simulink model "PMSM_realmodel"  (R2022b)
settings: Solver=FixedStepAuto  StartTime=0.0  StopTime=1  FixedStep=1e-6  MaxStep=1e-3  RelTol=1e-3
values from neighbouring files (symbols this model uses):
  a_fw = log(9)/trfw    [emrax_sim.m]
  ba = 2*k^2*(as*J - bm)/(np^2*psi)    [emrax_sim.m]
  bm = 0.008    [emrax_sim.m]
  fsw = 8e3    (= 8000)    [emrax_sim.m]
  I_max = I_base    [emrax_sim.m]
  J = 421e-4    (= 0.0421)    [emrax_sim.m]
  k = 1    [emrax_sim.m]
  ki_d = (ac^2)*Ld    [emrax_sim.m]
  ki_q = (ac^2)*Lq    [emrax_sim.m]
  ki_s = 2*k^2*as^2*J/(np^2*psi)    [emrax_sim.m]
  kp_d = ac*Ld    [emrax_sim.m]
  kp_q = ac*Lq    [emrax_sim.m]
  kp_s = 2*k^2*as*J/(np^2*psi)    [emrax_sim.m]
  Ld = 177*10^(-6)    (= 0.000177)    [emrax_sim.m]
  Lq = 183*10^(-6)    (= 0.000183)    [emrax_sim.m]
  np = 10    [emrax_sim.m]
  Peak_power = 50000    [emrax_sim.m]
  Peak_regen = -1500000    [emrax_sim.m]
  psi = 0.0542*k    (= 0.0542)    [emrax_sim.m]
  Ra_d = ac*Ld-Rs    [emrax_sim.m]
  Ra_q = ac*Lq-Rs    [emrax_sim.m]
  rpm_nom = 5100    [emrax_sim.m]
  Rs = 18e-3    (= 0.018)    [emrax_sim.m]
  u_dc = 550    [emrax_sim.m]
  u_nom = u_dc*k    (= 550)    [emrax_sim.m]
undefined symbols (not defined in the file or in its folder): Icutoff, rc1, rc2, rc3, rc4, rc5
libraries: simulink x9, spsIGBTDiodeLib x6, dspstat3 x3, spsCurrentMeasurementLib x3, spsSeriesRLCBranchLib x3, spsDCVoltageSourceLib x1, spsPermanentMagnetSynchronousMachineLib x1, spsThreePhaseVIMeasurementLib x1, spsMultimeterLib x1, spsTriangleGeneratorLib x1, sps_lib x1
settings Model: Creator=Vaggelis  LastModifiedBy=alexa
settings SolverCC: AlgebraicLoopSolver=TrustRegion
settings DebuggingCC: UnconnectedInputMsg=warning  UnconnectedOutputMsg=warning  UnconnectedLineMsg=warning  ArithmeticOperatorsInVariantConditions=warning
settings ModelReferenceCC: EnableRefExpFcnMdlSchedulingChecks=on
settings SFSimCC: CustomCodeUndefinedFunction=UseInterfaceOnly
settings RTWCC: DLArmComputeVersion=19.05

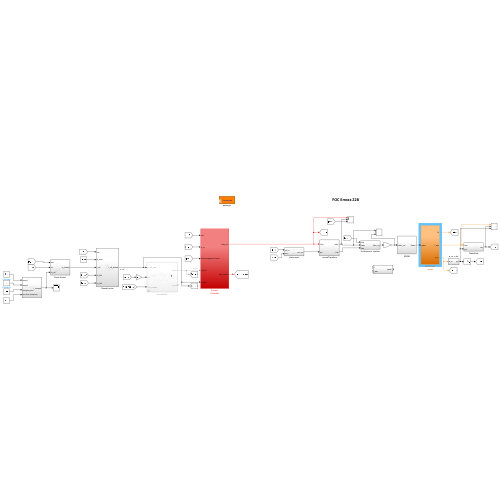
[thumbnail: Simulink's stored preview of the top-level diagram]
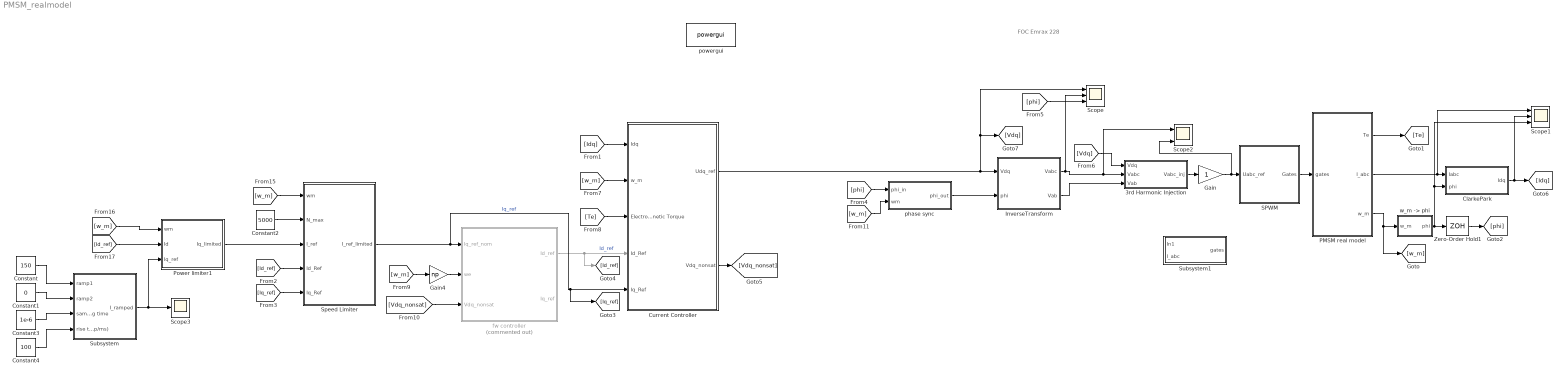
== system PMSM_realmodel ==
  note: FOC Emrax 228
  3rd Harmonic Injection : Subsystem
  ClarkePark : Subsystem
  Constant : Constant  Value=150
  Constant1 : Constant  Value=0
  Constant2 : Constant  Value=5000
  Constant3 : Constant  Value=1e-6
  Constant4 : Constant  Value=100
  Current Controller : Subsystem
  Gain : Gain
  Gain4 : Gain  Gain=np
  InverseTransform : Subsystem
  PMSM real model : Subsystem
  Power limiter1 : Subsystem
  SPWM : Subsystem
  Scope : Scope  NumInputPorts=3
  Scope1 : Scope  NumInputPorts=3
  Scope2 : Scope  NumInputPorts=3
  Scope3 : Scope
  Speed Limiter : Subsystem
  Subsystem : Subsystem
  Subsystem1 : Subsystem
  Zero-Order Hold1 : ZeroOrderHold  SampleTime=62e-6
  fw controller : Subsystem  Commented=on
  phase sync : Subsystem
  powergui : sps_lib/powergui  Priority=1  SimulationMode=Continuous  SampleTime=50e-6  frequency=60  Iterations=50  frequencyindice=0  Pbase=100e6  ErrMax=1e-4  UnitsV=kV  UnitsW=MW  buscounter=0  FunctionMessages=off  echomessages=off  EnableUseOfTLC=off  CurrentSourceSwitches=off  DisableSnubberDevices=off  DisableRonSwitches=off  DisableVfSwitches=off  DisplayEquations=off  AutomaticDiscreteSolvers=off  SolverType=Tustin/Backward Euler (TBE)  Interpol=off  ExternalGateDelay=off  methode=off  Ts=100  x0status=blocks  SPID=on  SwTol=0  HookPort=off  NonlinearTolerance=0  nMaxIteration=15  ContinueOnMaxIteration=off  RestoreLinks=warning  ResistiveCurrentMeasurement=off  Frange=[0:2:500]  Ylog=off  Xlog=on  ShowGrid=off  save=off  variable=ZData  structure=0  ZoomFFT=off  StartTime=0.0  cycles=1  DisplayStyle=1  fundamental=60  FreqAxis=off  MaxFrequency=1000  frequencyindicesteady=1  RmsSteady=1  display=off
  "w_m -> phi" : Subsystem
  wires:
  PMSM real model/3(w_m) -> [w_m], "w_m -> phi"/1(w_m)
  PMSM real model/1(Te) -> [Te]
  SPWM/1(Gates) -> PMSM real model/1("gates ")
  [Te] -> Current Controller/3(Electromagnetic Torque)
  Power limiter1/1(Iq_limited) -> Speed Limiter/3(I_ref)
  [w_m] -> Current Controller/2(w_m)
  [Iq_ref] -> Speed Limiter/5(Iq_Ref)
  [w_m] -> Gain4/1
  Constant2/1 -> Speed Limiter/2(N_max)
  [Id_ref] -> Power limiter1/2(Id)
  [Idq] -> Current Controller/1(Idq)
  [w_m] -> Power limiter1/1(wm)
  fw controller/1(Id_ref) -> [Id_ref], Current Controller/4(Id_Ref)  "Id_ref"
  Gain4/1 -> fw controller/2(we)
  [w_m] -> Speed Limiter/1(wm)
  Current Controller/2(Vdq_nonsat) -> [Vdq_nonsat]
  [Vdq_nonsat] -> fw controller/3(Vdq_nonsat)
  [Id_ref] -> Speed Limiter/4(Id_Ref)
  "w_m -> phi"/1(phi) -> ClarkePark/2(phi), Scope1/3, Zero-Order Hold1/1
  PMSM real model/2(I_abc) -> Scope1/1, ClarkePark/1(Iabc)
  ClarkePark/1(Idq) -> Scope1/2, [Idq]
  [phi] -> Scope/3
  Current Controller/1("Udq_ref ") -> Scope/1, [Vdq], InverseTransform/1(Vdq)
  3rd Harmonic Injection/1(Vabc_inj) -> Gain/1
  InverseTransform/1(Vabc) -> Scope/2, Scope2/1, 3rd Harmonic Injection/2(Vabc)
  [Vdq] -> 3rd Harmonic Injection/1(Vdq)
  InverseTransform/2(Vab) -> 3rd Harmonic Injection/3(Vab)
  Gain/1 -> SPWM/1(Uabc_ref), Scope2/3
  [phi] -> phase sync/1(phi_in)
  [w_m] -> phase sync/2(wm)
  phase sync/1(phi_out) -> InverseTransform/2(phi)
  Subsystem/1(I_ramped) -> Power limiter1/3(Iq_ref), Scope3/1
  Constant/1 -> Subsystem/1(ramp1)
  Constant1/1 -> Subsystem/2(ramp2)
  Constant3/1 -> Subsystem/3(sampling time)
  Constant4/1 -> Subsystem/4(rise time (Amp/ms))
  Zero-Order Hold1/1 -> [phi]
  Speed Limiter/1(I_ref_limited) -> [Iq_ref], Current Controller/5(Iq_Ref), fw controller/1(Iq_ref_nom)  "Iq_ref"

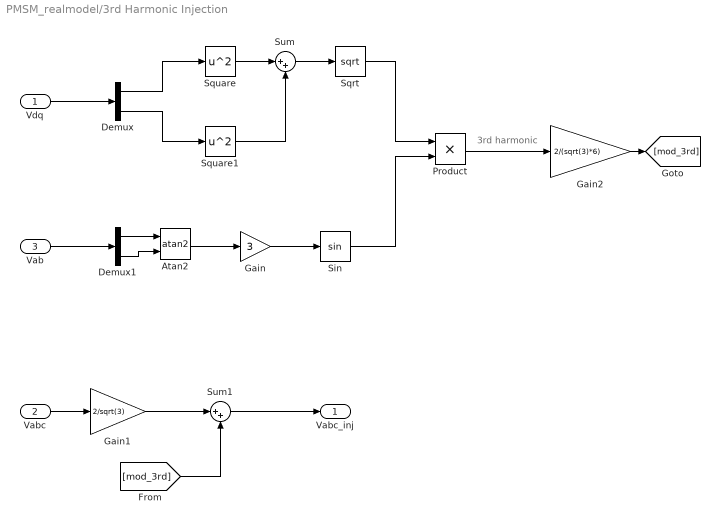
== system PMSM_realmodel/3rd Harmonic Injection ==
  note: 3rd harmonic
  Vdq : Inport
  Vabc : Inport  Port=2
  Vab : Inport  Port=3
  Atan2 : Trigonometry  Operator=atan2
  Demux : Demux  Outputs=2
  Demux1 : Demux  Outputs=2
  Gain : Gain  Gain=3
  Gain1 : Gain  Gain=2/sqrt(3)
  Gain2 : Gain  Gain=2/(sqrt(3)*6)
  Product : Product
  Sin : Trigonometry
  Sqrt : Sqrt
  Square : Math  Operator=square
  Square1 : Math  Operator=square
  Sum : Sum  Inputs=|++
  Sum1 : Sum  Inputs=|++
  Vabc_inj : Outport
  wires:
  Vdq/1 -> Demux/1
  Demux/1 -> Square/1
  Demux/2 -> Square1/1
  Square/1 -> Sum/1
  Square1/1 -> Sum/2
  Sum/1 -> Sqrt/1
  Vab/1 -> Demux1/1
  Demux1/1 -> Atan2/1
  Demux1/2 -> Atan2/2
  Atan2/1 -> Gain/1
  Gain/1 -> Sin/1
  Sqrt/1 -> Product/1
  Sin/1 -> Product/2
  Vabc/1 -> Gain1/1
  Product/1 -> Gain2/1
  Gain2/1 -> [mod_3rd]
  Gain1/1 -> Sum1/1
  [mod_3rd] -> Sum1/2
  Sum1/1 -> Vabc_inj/1

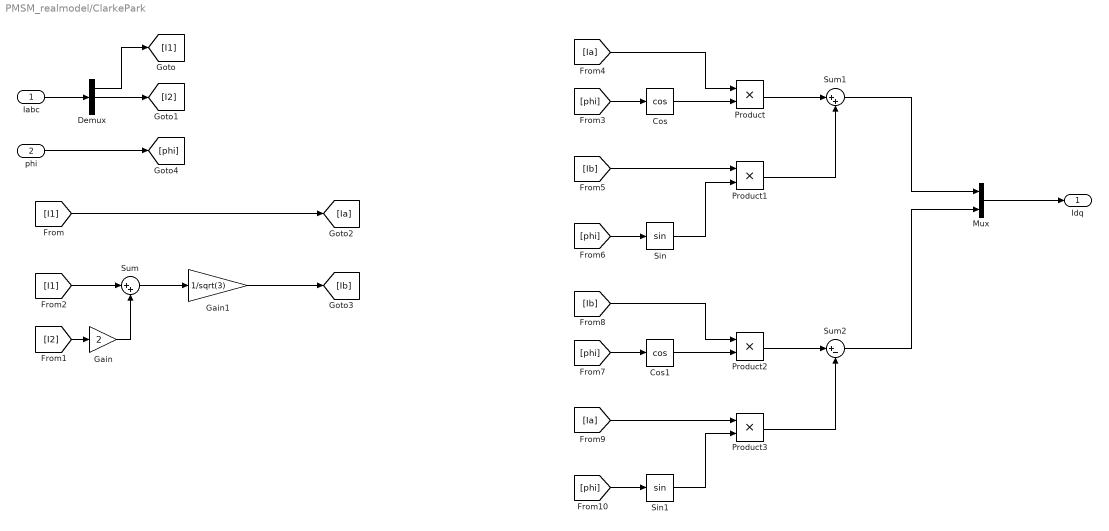
== system PMSM_realmodel/ClarkePark ==
  Iabc : Inport
  phi : Inport  Port=2
  Cos : Trigonometry  Operator=cos
  Cos1 : Trigonometry  Operator=cos
  Demux : Demux  Outputs=3
  Gain : Gain  Gain=2
  Gain1 : Gain  Gain=1/sqrt(3)
  Mux : Mux  Inputs=2
  Product{,1..3} (4 alike) : Product
  Sin : Trigonometry
  Sin1 : Trigonometry
  Sum : Sum  Inputs=|++
  Sum1 : Sum  Inputs=|++
  Sum2 : Sum  Inputs=|+-
  Idq : Outport
  wires:
  Iabc/1 -> Demux/1
  Demux/1 -> [I1]
  Demux/2 -> [I2]
  [I1] -> [Ia]
  [I1] -> Sum/1
  [I2] -> Gain/1
  Gain/1 -> Sum/2
  Sum/1 -> Gain1/1
  Gain1/1 -> [Ib]
  phi/1 -> [phi]
  [phi] -> Cos/1
  Cos/1 -> Product/2
  [Ia] -> Product/1
  Product/1 -> Sum1/1
  [phi] -> Sin/1
  [Ib] -> Product1/1
  Sin/1 -> Product1/2
  Product1/1 -> Sum1/2
  Sum1/1 -> Mux/1
  Mux/1 -> Idq/1
  Product3/1 -> Sum2/2
  Sin1/1 -> Product3/2
  [Ia] -> Product3/1
  [phi] -> Sin1/1
  Product2/1 -> Sum2/1
  [Ib] -> Product2/1
  Cos1/1 -> Product2/2
  [phi] -> Cos1/1
  Sum2/1 -> Mux/2

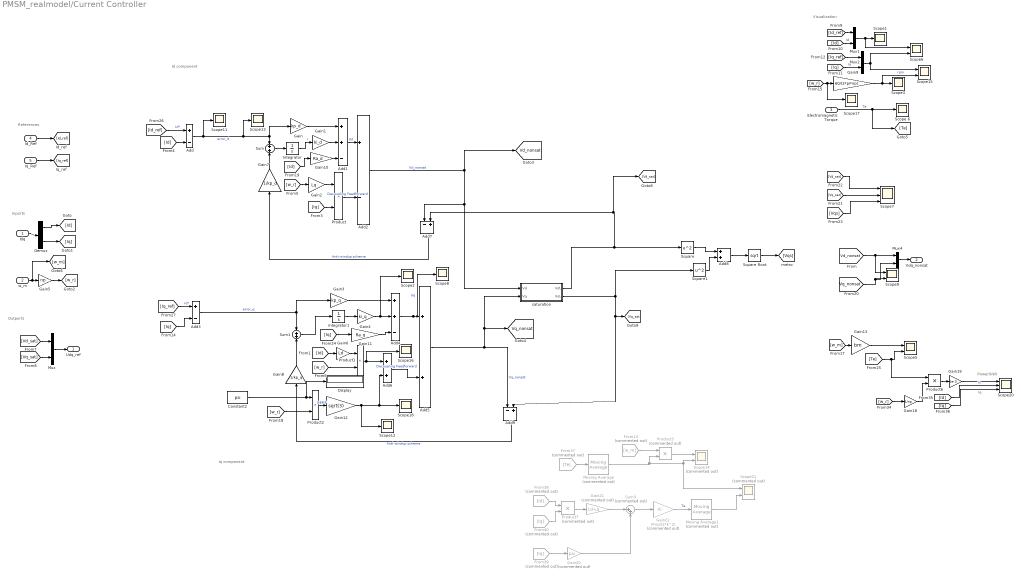
== system PMSM_realmodel/Current Controller ==
  note: References
  note: Id component
  note: Iq component
  note: Inports
  note: Outports
  note: Visualization
  note: Power(kW)
  Idq : Inport
  w_m : Inport  Port=2
  Electromagnetic Torque : Inport  Port=3
  Id_Ref : Inport  Port=4
  Iq_Ref : Inport  Port=5
  Add : Sum  Inputs=+-
  Add1 : Sum  Inputs=++-
  Add2 : Sum  Inputs=+-
  Add3 : Sum  Inputs=+-
  Add4 : Sum  Inputs=++-
  Add5 : Sum
  Add6 : Sum
  Add7 : Sum  Inputs=-+
  Add8 : Sum
  Add9 : Sum  Inputs=-+
  Constant2 : Constant  Value=psi
  Demux : Demux  Outputs=2
  Display : Display
  From13 : From  Commented=on  GotoTag=w_m
  From37 : From  Commented=on  GotoTag=Te
  From38 : From  Commented=on  GotoTag=Id
  From39 : From  Commented=on  GotoTag=Iq
  From40 : From  Commented=on  GotoTag=Iq
  Gain : Gain  Gain=kp_d
  Gain1 : Gain  Gain=ki_d
  Gain10 : Gain  Gain=Ra_d
  Gain11 : Gain  Gain=Ra_q
  Gain12 : Gain  Gain=sqrt(3)
  Gain13 : Gain  Gain=bm
  Gain18 : Gain  Gain=1/np
  Gain19 : Gain  Gain=1e-3
  Gain2 : Gain  Gain=Lq
  Gain20 : Gain  Commented=on  Gain=psi
  Gain21 : Gain  Commented=on  Gain=Ld-Lq
  Gain22 : Gain  Commented=on  Gain=3*np/(2*k^2)
  Gain3 : Gain  Gain=kp_q
  Gain4 : Gain  Gain=ki_q
  Gain5 : Gain  Gain=np
  Gain6 : Gain  Gain=Ld
  Gain7 : Gain  Gain=1/kp_d
  Gain8 : Gain  Gain=1/kp_q
  Gain9 : Gain  Gain=60/(2*pi*np)
  Integrator : Integrator
  Integrator1 : Integrator
  Moving Average : dspstat3/Moving Average  Commented=on  Method=Sliding window  ForgettingFactorPort=off  SpecifyWindowLength=on  WindowLength=40000  OverlapLength=39999  AllowArbitraryInputLength=off  ForgettingFactor=0.9  SimulateUsing=Code generation
  Moving Average1 : dspstat3/Moving Average  Commented=on  Method=Sliding window  ForgettingFactorPort=off  SpecifyWindowLength=on  WindowLength=40000  OverlapLength=39999  AllowArbitraryInputLength=off  ForgettingFactor=0.9  SimulateUsing=Code generation
  Mux{,1..2,4} (4 alike) : Mux  Inputs=2
  Product{,1..2,6} (4 alike) : Product
  Product3 : Product  Commented=on
  Product7 : Product  Commented=on
  Scope 6 : Scope
  Scope{1..3,8,11..13,16..18} (10 alike) : Scope
  Scope14 : Scope  Commented=on  NumInputPorts=2
  Scope{5..6,9,15} (4 alike) : Scope  NumInputPorts=2
  Scope20 : Scope  NumInputPorts=3
  Scope21 : Scope  Commented=on  NumInputPorts=2
  Scope7 : Scope  NumInputPorts=3
  Square : Math  Operator=square
  Square Root : Sqrt
  Square1 : Math  Operator=square
  Sum : Sum
  Sum1 : Sum
  Sum3 : Sum  Commented=on  Inputs=|++
  saturation : Subsystem
  "Udq_ref " : Outport  VectorParamsAs1DForOutWhenUnconnected=off
  Vdq_nonsat : Outport  Port=2
  tag scope: Vd_nonsat=global, Vq_nonsat=global
  wires:
  Gain4/1 -> Scope2/1, Add4/2
  [Id] -> Gain6/1
  Add4/1 -> Scope8/1, Add5/1  "Uq"
  Add1/1 -> Add2/1  "Ud"
  [w_r] -> Gain2/1
  Gain2/1 -> Product/1
  Gain3/1 -> Add4/1
  [Iq] -> Product/2
  Integrator/1 -> Gain1/1  "I"
  Sum/1 -> Integrator/1
  Gain/1 -> Add1/1
  [w_r] -> Product1/2
  Gain6/1 -> Product1/1
  Idq/1 -> Demux/1
  Product/1 -> Add2/2  "Decoupling Feedforward"
  Gain7/1 -> Sum/2
  Add2/1 -> [Vd_nonsat], saturation/1(Vd), Add7/1  "Vd_nonsat"
  Add7/1 -> Gain7/1  "Anti-windup scheme"
  Sum1/1 -> Integrator1/1
  Add5/1 -> Add9/1, saturation/2(Vq), [Vq_nonsat]  "Vq_nonsat"
  Gain8/1 -> Sum1/2
  Add9/1 -> Gain8/1  "Anti-windup scheme"
  Demux/1 -> [Id]
  Demux/2 -> [Iq]
  w_m/1 -> [w_m], Gain5/1
  Gain5/1 -> [w_r]
  [Vd_sat] -> Mux/1
  [Vq_sat] -> Mux/2
  Mux/1 -> "Udq_ref "/1
  [Id] -> Add/2
  Mux1/1 -> Scope6/1, Scope1/1
  [Id_ref] -> Mux1/1
  [Id] -> Mux1/2  "Id"
  [Iq_ref] -> Mux2/1
  [Iq] -> Mux2/2  "Iq"
  [w_r] -> Scope17/1, Gain9/1
  Gain9/1 -> Scope15/2, Scope3/1  "rpm"
  Electromagnetic Torque/1 -> Scope 6/1, [Te]  "Te"
  Product1/1 -> Scope16/1, Add6/1
  Add6/1 -> Add5/2  "Decoupling Feedforward"
  Add/1 -> Scope13/1, Sum/1, Gain/1, Scope11/1  "error_d"
  Add3/1 -> Sum1/1, Gain3/1  "error_q"
  [Iq] -> Add3/2
  Gain1/1 -> Add1/2
  Integrator1/1 -> Gain4/1
  Square1/1 -> Add8/2
  Square/1 -> Add8/1
  Add8/1 -> Square Root/1
  [Vd_nonsat] -> Scope9/1, Mux4/1
  [Vq_nonsat] -> Mux4/2, Scope9/2
  Square Root/1 -> [Vqs]
  [Vd_sat] -> Scope7/1
  [Vq_sat] -> Scope7/2
  [Vqs] -> Scope7/3
  [Id] -> Gain10/1
  [Iq] -> Gain11/1
  Id_Ref/1 -> [Id_ref]
  Iq_Ref/1 -> [Iq_ref]
  Gain13/1 -> Scope5/1
  [Te] -> Product6/1, Scope5/2
  [w_m] -> Gain13/1
  Mux2/1 -> Scope6/2, Scope15/1
  [Id_ref] -> Add/1  "Id*"
  saturation/1(Vd\) -> Square/1, [Vd_sat], Add7/2
  saturation/2(Vq\) -> Square1/1, [Vq_sat], Add9/2
  Gain10/1 -> Add1/3
  Gain11/1 -> Add4/3
  [w_r] -> Product2/2
  Product2/1 -> Gain12/1  "BEMF"
  Mux4/1 -> Vdq_nonsat/1
  [Iq_ref] -> Add3/1  "Id*"
  Gain19/1 -> Scope20/1
  [Iq] -> Scope20/3  "Iq"
  [Id] -> Scope20/2  "Id"
  Gain18/1 -> Product6/2
  Product6/1 -> Gain19/1
  [w_r] -> Gain18/1
  Constant2/1 -> Display/1, Product2/1
  Product3/1 -> Scope14/1
  From13/1 -> Product3/1
  Moving Average/1 -> Scope14/2, Scope21/1, Product3/2
  From37/1 -> Moving Average/1
  From39/1 -> Gain20/1
  Product7/1 -> Gain21/1
  From38/1 -> Product7/1
  From40/1 -> Product7/2
  Gain21/1 -> Sum3/1
  Gain20/1 -> Sum3/2
  Sum3/1 -> Gain22/1
  Gain22/1 -> Moving Average1/1  "Te"
  Moving Average1/1 -> Scope21/2
  Gain12/1 -> Scope12/1, Add6/2, Scope18/1

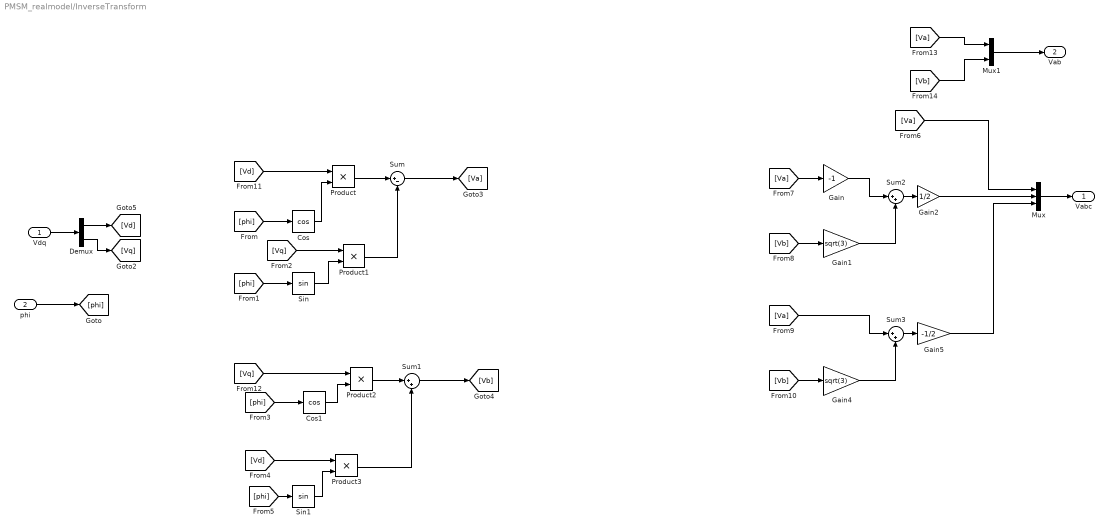
== system PMSM_realmodel/InverseTransform ==
  Vdq : Inport
  phi : Inport  Port=2
  Cos : Trigonometry  Operator=cos
  Cos1 : Trigonometry  Operator=cos
  Demux : Demux  Outputs=2
  Gain : Gain  Gain=-1
  Gain1 : Gain  Gain=sqrt(3)
  Gain2 : Gain  Gain=1/2
  Gain4 : Gain  Gain=sqrt(3)
  Gain5 : Gain  Gain=-1/2
  Mux : Mux  Inputs=3
  Mux1 : Mux  Inputs=2
  Product{,1..3} (4 alike) : Product
  Sin : Trigonometry
  Sin1 : Trigonometry
  Sum : Sum  Inputs=|+-
  Sum1 : Sum  Inputs=|++
  Sum2 : Sum  Inputs=|++
  Sum3 : Sum  Inputs=|++
  Vabc : Outport
  Vab : Outport  Port=2
  wires:
  phi/1 -> [phi]
  [phi] -> Cos/1
  Cos/1 -> Product/2
  Product/1 -> Sum/1
  [phi] -> Sin/1
  [Vq] -> Product1/1
  Sin/1 -> Product1/2
  Product1/1 -> Sum/2
  Cos1/1 -> Product2/2
  [phi] -> Cos1/1
  Product2/1 -> Sum1/1
  Sin1/1 -> Product3/2
  [phi] -> Sin1/1
  [Vd] -> Product3/1
  Product3/1 -> Sum1/2
  Sum/1 -> [Va]
  Sum1/1 -> [Vb]
  [Va] -> Mux/1
  [Va] -> Gain/1
  [Vb] -> Gain1/1
  Gain/1 -> Sum2/1
  Gain1/1 -> Sum2/2
  Sum2/1 -> Gain2/1
  Gain2/1 -> Mux/2
  Sum3/1 -> Gain5/1
  Gain4/1 -> Sum3/2
  [Va] -> Sum3/1
  [Vb] -> Gain4/1
  Vdq/1 -> Demux/1
  Demux/1 -> [Vd]
  Demux/2 -> [Vq]
  [Vd] -> Product/1
  [Vq] -> Product2/1
  Gain5/1 -> Mux/3
  Mux/1 -> Vabc/1
  Mux1/1 -> Vab/1
  [Va] -> Mux1/1
  [Vb] -> Mux1/2

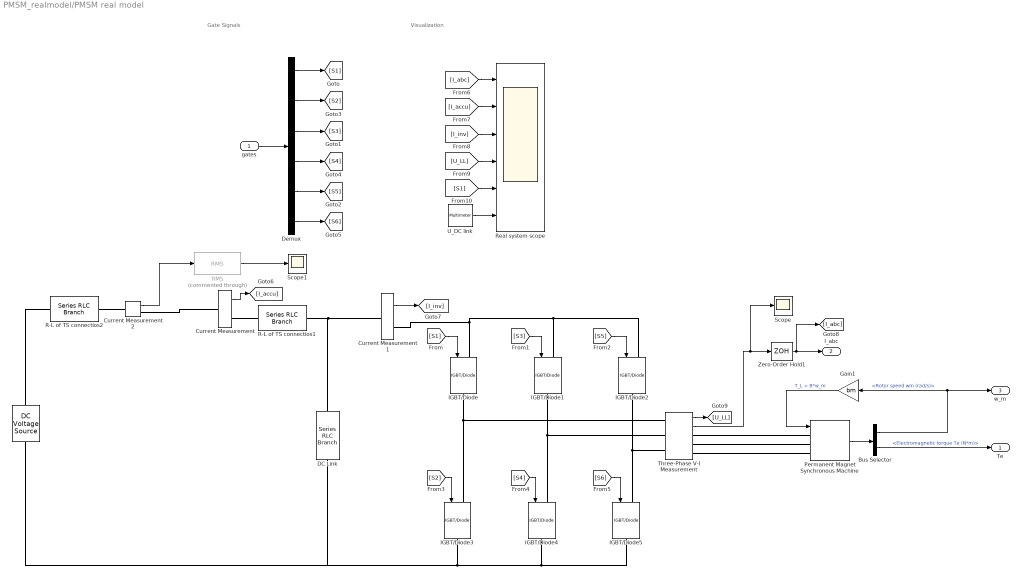
== system PMSM_realmodel/PMSM real model ==
  note: Gate Signals
  note: Visualization
  "gates " : Inport
  " " : spsDCVoltageSourceLib/DC Voltage Source  Description=source block  Amplitude=u_dc  Measurements=None
      settings: AttributesFormatString=\n
  Bus Selector : BusSelector  OutputSignals=Rotor speed wm (rad/s),Electromagnetic torque Te (N*m)
  Current Measurement : spsCurrentMeasurementLib/Current Measurement  PhasorSimulation=off  OutputType=Complex  PSBequivalent=0
  Current Measurement1 : spsCurrentMeasurementLib/Current Measurement  PhasorSimulation=off  OutputType=Complex  PSBequivalent=0
  Current Measurement2 : spsCurrentMeasurementLib/Current Measurement  PhasorSimulation=off  OutputType=Complex  PSBequivalent=0
  DC Link : spsSeriesRLCBranchLib/Series RLC Branch  LConnTagsString=__new0  RConnTagsString=__new0  BranchType=C  Resistance=1  Inductance=1e-3  SetiL0=off  InitialCurrent=0  Capacitance=700e-6  Setx0=off  InitialVoltage=0  Measurements=Branch voltage
  Demux : Demux  Outputs=6
  Gain1 : Gain  Gain=bm
  IGBT/Diode{,1..5} (6 alike) : spsIGBTDiodeLib/IGBT//Diode  Ron=1e-3  Rs=1e5  Cs=inf  Measurements=off
  Permanent Magnet Synchronous Machine : spsPermanentMagnetSynchronousMachineLib/Permanent Magnet Synchronous Machine  NbPhases=3  FluxDistribution=Sinusoidal  RotorType=Salient-pole  MechanicalLoad=Torque Tm  PresetModel=No  ShowDetailedParameters=on  MeasurementBus=off  Resistance=Rs  Inductance=8.5e-3  dqInductances=[Ld Lq]  La=0.00153  MachineConstant=Flux linkage established by magnets (V.s)  Flux=psi  VoltageCst=98.3079  TorqueCst=0.813  Flat=120  Mechanical=[J 0 np 0]  PolePairs=4  InitialConditions=[0,0, 0,0]  InitialConditions5ph=[0 0 0 0 0 0]  RefAngle=Aligned with phase A axis (original Park)  IterativeDiscreteModel=Trapezoidal non iterative  TsBlock=-1  TsPowergui=0
  R-L of TS connectios1 : spsSeriesRLCBranchLib/Series RLC Branch  LConnTagsString=__new0  RConnTagsString=__new0  BranchType=RL  Resistance=20e-4  Inductance=1e-8  SetiL0=off  InitialCurrent=0  Capacitance=300e-6  Setx0=off  InitialVoltage=0  Measurements=None
  R-L of TS connectios2 : spsSeriesRLCBranchLib/Series RLC Branch  LConnTagsString=__new0  RConnTagsString=__new0  BranchType=RL  Resistance=86.4e-3  Inductance=1e-7  SetiL0=off  InitialCurrent=0  Capacitance=300e-6  Setx0=off  InitialVoltage=0  Measurements=None
  RMS : dspstat3/RMS  Commented=through  run=off  directionMode=Each column  dimension=1  InputProcessing=Columns as channels (frame based)  reset_popup=None
  Real system scope : Scope  NumInputPorts=6
  Scope : Scope
  Scope1 : Scope
  Three-Phase V-I Measurement : spsThreePhaseVIMeasurementLib/Three-Phase V-I Measurement  VoltageMeasurement=phase-to-phase  SetLabelV=off  LabelV=Vabc  Vpu=off  VpuLL=off  CurrentMeasurement=yes  SetLabelI=off  LabelI=Iabc  Ipu=off  Pbase=100e6  Vbase=500e3  OutputType=Complex  PhasorSimulation=off  PSBequivalent=0
  U_DC link : spsMultimeterLib/Multimeter  L=1  sel=1  yselected={}  Gain=1  OutputType=Complex  PlotAtSimulationStop=off  PhasorSimulation=off
  Zero-Order Hold1 : ZeroOrderHold  SampleTime=62e-6
  Te : Outport  VectorParamsAs1DForOutWhenUnconnected=off
  I_abc : Outport  Port=2  VectorParamsAs1DForOutWhenUnconnected=off
  w_m : Outport  Port=3  VectorParamsAs1DForOutWhenUnconnected=off
  wires:
  [S2] -> IGBT/Diode3/1
  [S3] -> IGBT/Diode1/1
  Gain1/1 -> Permanent Magnet Synchronous Machine/1  "T_L = B*w_m"
  [S1] -> IGBT/Diode/1
  [S6] -> IGBT/Diode5/1
  [S4] -> IGBT/Diode4/1
  [S5] -> IGBT/Diode2/1
  Permanent Magnet Synchronous Machine/1 -> Bus Selector/1
  Bus Selector/1 -> Gain1/1, w_m/1  "<Rotor speed wm (rad/s)>"
  Bus Selector/2 -> Te/1  "<Electromagnetic torque Te (N*m)>"
  "gates "/1 -> Demux/1
  Demux/1 -> [S1]
  Demux/2 -> [S2]
  Demux/3 -> [S3]
  Demux/4 -> [S4]
  Demux/5 -> [S5]
  Demux/6 -> [S6]
  Three-Phase V-I Measurement/2 -> Zero-Order Hold1/1, Scope/1
  Current Measurement/1 -> [I_accu]
  Current Measurement1/1 -> [I_inv]
  [I_abc] -> Real system scope/1
  [I_accu] -> Real system scope/2
  [I_inv] -> Real system scope/3
  Three-Phase V-I Measurement/1 -> [U_LL]
  [U_LL] -> Real system scope/4
  [S1] -> Real system scope/5
  U_DC link/1 -> Real system scope/6
  Zero-Order Hold1/1 -> I_abc/1, [I_abc]
  Current Measurement2/1 -> RMS/1
  RMS/1 -> Scope1/1
  connections:
  Three-Phase V-I Measurement/RConn2 -- Permanent Magnet Synchronous Machine/LConn2
  Current Measurement/RConn1 -- R-L of TS connectios1/RConn1
  IGBT/Diode2/RConn1 -- IGBT/Diode5/LConn1 -- Three-Phase V-I Measurement/LConn3
  IGBT/Diode1/RConn1 -- IGBT/Diode4/LConn1 -- Three-Phase V-I Measurement/LConn2
  Three-Phase V-I Measurement/RConn1 -- Permanent Magnet Synchronous Machine/LConn1
  IGBT/Diode/RConn1 -- Three-Phase V-I Measurement/LConn1 -- IGBT/Diode3/LConn1
  IGBT/Diode3/RConn1 -- " "/LConn1 -- DC Link/RConn1 -- IGBT/Diode4/RConn1 -- IGBT/Diode5/RConn1
  Three-Phase V-I Measurement/RConn3 -- Permanent Magnet Synchronous Machine/LConn3
  IGBT/Diode/LConn1 -- IGBT/Diode1/LConn1 -- IGBT/Diode2/LConn1 -- Current Measurement1/RConn1
  R-L of TS connectios1/LConn1 -- Current Measurement1/LConn1 -- DC Link/LConn1
  R-L of TS connectios2/RConn1 -- " "/RConn1
  Current Measurement2/LConn1 -- R-L of TS connectios2/LConn1
  Current Measurement2/RConn1 -- Current Measurement/LConn1

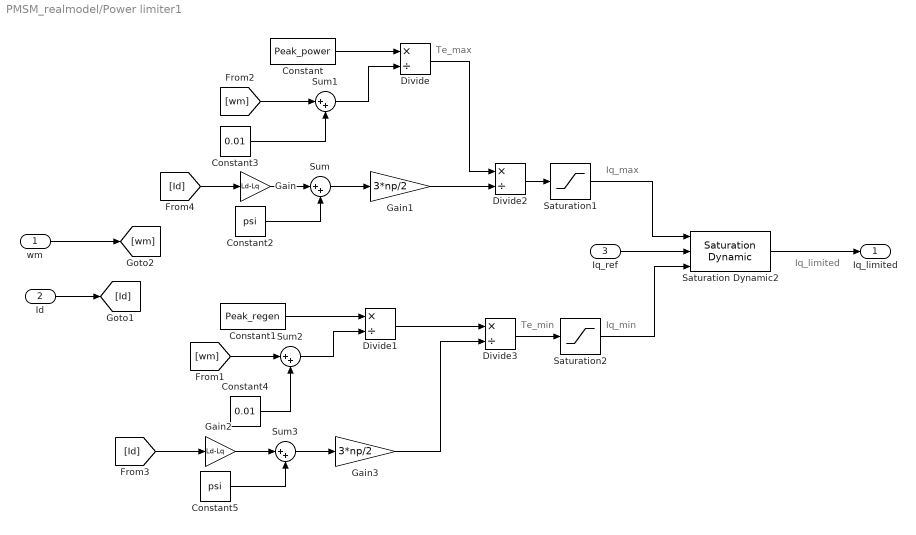
== system PMSM_realmodel/Power limiter1 ==
  note: Te_max
  note: Iq_limited
  note: Iq_max
  note: Iq_min
  note: Te_min
  wm : Inport
  Id : Inport  Port=2
  Iq_ref : Inport  Port=3
  Constant : Constant  Value=Peak_power
  Constant1 : Constant  Value=Peak_regen
  Constant2 : Constant  Value=psi
  Constant3 : Constant  Value=0.01
  Constant4 : Constant  Value=0.01
  Constant5 : Constant  Value=psi
  Divide{,1..3} (4 alike) : Product  Inputs=*/
  Gain : Gain  Gain=Ld-Lq
  Gain1 : Gain  Gain=3*np/2
  Gain2 : Gain  Gain=Ld-Lq
  Gain3 : Gain  Gain=3*np/2
  Saturation Dynamic2 : simulink/Discontinuities/Saturation Dynamic  OutMin=[]  OutMax=[]  OutDataTypeStr=Inherit: Same as second input  OutDataType=fixdt(1, 16)  OutScaling=2^-10  DoSatur=off
  Saturation1 : Saturate  UpperLimit=10000  LowerLimit=-10000
  Saturation2 : Saturate  UpperLimit=10000  LowerLimit=-10000
  Sum{,1..3} (4 alike) : Sum  Inputs=|++
  Iq_limited : Outport
  wires:
  Sum2/1 -> Divide1/2
  [wm] -> Sum2/1
  Constant4/1 -> Sum2/2
  Saturation2/1 -> Saturation Dynamic2/3
  Saturation1/1 -> Saturation Dynamic2/1
  Constant3/1 -> Sum1/2
  [wm] -> Sum1/1
  Sum1/1 -> Divide/2
  Divide2/1 -> Saturation1/1
  Divide3/1 -> Saturation2/1
  Divide/1 -> Divide2/1
  Constant1/1 -> Divide1/1
  Constant/1 -> Divide/1
  Divide1/1 -> Divide3/1
  Saturation Dynamic2/1 -> Iq_limited/1
  wm/1 -> [wm]
  Iq_ref/1 -> Saturation Dynamic2/2
  Gain1/1 -> Divide2/2
  Gain/1 -> Sum/1
  Constant2/1 -> Sum/2
  Sum/1 -> Gain1/1
  Sum3/1 -> Gain3/1
  [Id] -> Gain2/1
  Gain2/1 -> Sum3/1
  Constant5/1 -> Sum3/2
  Gain3/1 -> Divide3/2
  Id/1 -> [Id]
  [Id] -> Gain/1

== system PMSM_realmodel/SPWM ==
  Uabc_ref : Inport
  Add : Sum  Inputs=+-
  Add1 : Sum  Inputs=+-
  Add2 : Sum  Inputs=+-
  Compare To Zero : simulink/Logic and Bit Operations/Compare To Zero  relop=>=  OutDataTypeStr=boolean  ZeroCross=off
  Compare To Zero1 : simulink/Logic and Bit Operations/Compare To Zero  relop=>=  OutDataTypeStr=boolean  ZeroCross=off
  Compare To Zero2 : simulink/Logic and Bit Operations/Compare To Zero  relop=>=  OutDataTypeStr=boolean  ZeroCross=off
  Delay1 : Delay  DelayLength=62  InitialCondition=0  UseCircularBuffer=on
  Demux : Demux  Outputs=3
  Gain : Gain  Gain=1/u_dc
  Mux : Mux  Inputs=6
  NOT : Logic  Operator=NOT  IconShape=distinctive  AllPortsSameDT=off  OutDataTypeStr=boolean
  NOT1 : Logic  Operator=NOT  IconShape=distinctive  AllPortsSameDT=off  OutDataTypeStr=boolean
  NOT2 : Logic  Operator=NOT  IconShape=distinctive  AllPortsSameDT=off  OutDataTypeStr=boolean
  Scope : Scope  NumInputPorts=2
  Scope1 : Scope  NumInputPorts=3
  Triangle Generator1 : spsTriangleGeneratorLib/Triangle Generator  Freq=fsw  Phase=90  Ts=1e-6
  Zero-Order Hold : ZeroOrderHold  SampleTime=62e-6
  Gates : Outport  VectorParamsAs1DForOutWhenUnconnected=off
  wires:
  Triangle Generator1/1 -> Add/2, Add2/2, Add1/2, Scope/1
  Add/1 -> Compare To Zero/1
  Compare To Zero/1 -> NOT/1, Mux/1
  Add2/1 -> Compare To Zero2/1
  Compare To Zero1/1 -> Mux/3, NOT1/1
  Compare To Zero2/1 -> Mux/5, NOT2/1
  NOT1/1 -> Mux/4
  Demux/1 -> Scope/2, Add/1
  NOT2/1 -> Mux/6
  Gain/1 -> Scope1/1, Delay1/1  "scale for triangle  comparison"
  Add1/1 -> Compare To Zero1/1
  Demux/2 -> Add1/1
  Uabc_ref/1 -> Gain/1
  Demux/3 -> Add2/1
  NOT/1 -> Mux/2
  Mux/1 -> Gates/1
  Zero-Order Hold/1 -> Scope1/3, Demux/1
  Delay1/1 -> Scope1/2, Zero-Order Hold/1

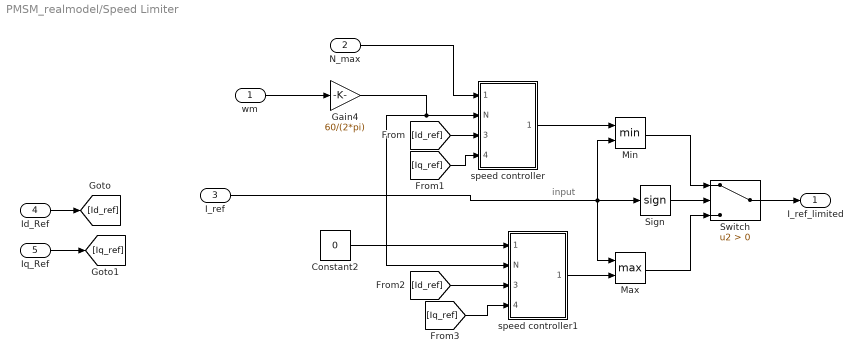
== system PMSM_realmodel/Speed Limiter ==
  note: input
  wm : Inport
  N_max : Inport  Port=2
  I_ref : Inport  Port=3
  Id_Ref : Inport  Port=4
  Iq_Ref : Inport  Port=5
  Constant2 : Constant  Value=0
  Gain4 : Gain  Gain=60/(2*pi)
  Max : MinMax  Function=max  Inputs=2
  Min : MinMax  Inputs=2
  Sign : Signum
  Switch : Switch  Criteria=u2 > Threshold  SaturateOnIntegerOverflow=off  InputSameDT=off
  speed controller : Subsystem
  speed controller1 : Subsystem
  I_ref_limited : Outport
  wires:
  speed controller1/1(Iq_ref) -> Max/2
  Max/1 -> Switch/3
  [Id_ref] -> speed controller1/3(Id_ref)
  I_ref/1 -> Max/1, Sign/1, Min/2
  [Iq_ref] -> speed controller/4(Iq_ref_sat)
  [Id_ref] -> speed controller/3(Id_ref)
  [Iq_ref] -> speed controller1/4(Iq_ref_sat)
  speed controller/1(Iq_ref) -> Min/1
  Gain4/1 -> speed controller/2(N), speed controller1/2(N)
  N_max/1 -> speed controller/1(N_ref)
  Constant2/1 -> speed controller1/1(N_ref)
  Min/1 -> Switch/1
  Sign/1 -> Switch/2
  wm/1 -> Gain4/1
  Switch/1 -> I_ref_limited/1
  Id_Ref/1 -> [Id_ref]
  Iq_Ref/1 -> [Iq_ref]

== system PMSM_realmodel/Subsystem ==
  ramp1 : Inport
  ramp2 : Inport  Port=2
  sampling time : Inport  Port=3
  rise time (Amp/ms) : Inport  Port=4
  Constant5 : Constant  Value=0
  Gain : Gain  Gain=1000
  Gain1 : Gain  Gain=0.1
  Memory1 : Memory
  Memory2 : Memory
  Product : Product
  Product1 : Product
  Saturation Dynamic1 : simulink/Discontinuities/Saturation Dynamic  OutMin=[]  OutMax=[]  OutDataTypeStr=Inherit: Same as second input  OutDataType=fixdt(1, 16)  OutScaling=2^-10  DoSatur=off
  Step3 : Step  Time=0.4  Before=1  After=-1  SampleTime=0
  Sum1 : Sum  Inputs=|+++
  Sum4 : Sum  Inputs=|-+
  Switch1 : Switch  Criteria=u2 > Threshold  SaturateOnIntegerOverflow=off  InputSameDT=off
  Switch2 : Switch  Criteria=u2 > Threshold  SaturateOnIntegerOverflow=off  InputSameDT=off
  I_ramped : Outport
  wires:
  Sum1/1 -> Memory2/1, Sum4/1, Memory1/1, Saturation Dynamic1/2
  Switch2/1 -> Product1/2
  Memory2/1 -> Switch2/2
  Product1/1 -> Sum1/1
  Memory1/1 -> Sum1/3
  Gain1/1 -> Switch2/3
  Switch1/1 -> Saturation Dynamic1/3
  Step3/1 -> Switch1/2, Product1/1  "Id*"
  Sum4/1 -> Sum1/2
  Constant5/1 -> Switch1/1
  Saturation Dynamic1/1 -> Sum4/2, I_ramped/1
  ramp2/1 -> Switch1/3
  ramp1/1 -> Saturation Dynamic1/1
  rise time (Amp/ms)/1 -> Gain/1
  sampling time/1 -> Product/2
  Gain/1 -> Product/1
  Product/1 -> Switch2/1, Gain1/1

== system PMSM_realmodel/Subsystem1 ==
  In1 : Inport
  I_abc : Inport  Port=2
  Constant : Constant  Value=200
  Constant5 : Constant  Value=0
  Demux : Demux  Outputs=3
  Demux1 : Demux  Outputs=3
  Scope : Scope  NumInputPorts=2
  Switch : Switch  Criteria=u2 > Threshold  Threshold=Icutoff  SaturateOnIntegerOverflow=off  InputSameDT=off
  Switch1 : Switch  Criteria=u2 > Threshold  Threshold=Icutoff  SaturateOnIntegerOverflow=off  InputSameDT=off
  Switch2 : Switch  Criteria=u2 > Threshold  Threshold=Icutoff  SaturateOnIntegerOverflow=off  InputSameDT=off
  Transfer Fcn : TransferFcn  Numerator=[rc1]  Denominator=[1 rc1]
  Transfer Fcn1 : TransferFcn  Numerator=[rc2]  Denominator=[1 rc2]
  Transfer Fcn2 : TransferFcn  Numerator=[rc3]  Denominator=[1 rc3]
  Transfer Fcn3 : TransferFcn  Numerator=[rc4]  Denominator=[1 rc4]
  Transfer Fcn4 : TransferFcn  Numerator=[rc5]  Denominator=[1 rc5]
  Transport Delay : TransportDelay  DelayTime=1e-6
  "gates " : Outport
  wires:
  Transfer Fcn/1 -> Transfer Fcn1/1
  I_abc/1 -> Demux/1
  Switch2/1 -> Transfer Fcn/1
  Demux/1 -> Switch2/3
  Constant/1 -> Switch2/1
  Constant5/1 -> Switch/1
  In1/1 -> Switch/3
  Transfer Fcn1/1 -> Transfer Fcn2/1
  Switch/1 -> "gates "/1
  Transport Delay/1 -> Switch2/2, Switch/2
  Transfer Fcn2/1 -> Transfer Fcn3/1
  Transfer Fcn3/1 -> Transfer Fcn4/1
  Transfer Fcn4/1 -> Transport Delay/1

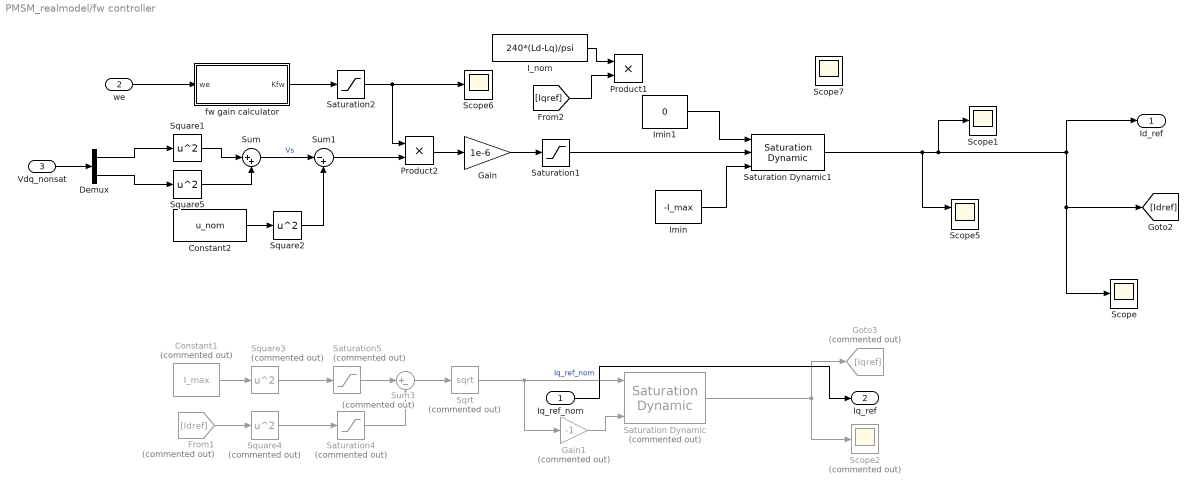
== system PMSM_realmodel/fw controller ==
  Iq_ref_nom : Inport
  we : Inport  Port=2
  Vdq_nonsat : Inport  Port=3
  Constant1 : Constant  Commented=on  Value=I_max
  Constant2 : Constant  Value=u_nom
  Demux : Demux  Outputs=2
  From1 : From  Commented=on  GotoTag=Idref
  Gain : Gain  Gain=1e-6
  Gain1 : Gain  Commented=on  Gain=-1
  Goto3 : Goto  Commented=on  GotoTag=Iqref
  I_nom : Constant  Value=240*(Ld-Lq)/psi
  Imin : Constant  Value=-I_max
  Imin1 : Constant  Value=0
  Product1 : Product
  Product2 : Product
  Saturation Dynamic : simulink/Discontinuities/Saturation Dynamic  Commented=on  OutMin=[]  OutMax=[]  OutDataTypeStr=Inherit: Same as second input  OutDataType=fixdt(1, 16)  OutScaling=2^-10  DoSatur=off
  Saturation Dynamic1 : simulink/Discontinuities/Saturation Dynamic  OutMin=[]  OutMax=[]  OutDataTypeStr=Inherit: Same as second input  OutDataType=fixdt(1, 16)  OutScaling=2^-10  DoSatur=off
  Saturation1 : Saturate  UpperLimit=150  LowerLimit=-150
  Saturation2 : Saturate  UpperLimit=5  LowerLimit=-5
  Saturation4 : Saturate  Commented=on  UpperLimit=10000  LowerLimit=-1000000
  Saturation5 : Saturate  Commented=on  UpperLimit=10000  LowerLimit=-1000000
  Scope{,1,6..7} (4 alike) : Scope
  Scope2 : Scope  Commented=on
  Scope5 : Scope  NumInputPorts=2
  Sqrt : Sqrt  Commented=on
  Square1 : Math  Operator=square
  Square2 : Math  Operator=square
  Square3 : Math  Commented=on  Operator=square
  Square4 : Math  Commented=on  Operator=square
  Square5 : Math  Operator=square
  Sum : Sum  Inputs=|++
  Sum1 : Sum  Inputs=|-+
  Sum3 : Sum  Commented=on  Inputs=|+-
  fw gain calculator : Subsystem
  Id_ref : Outport
  Iq_ref : Outport  Port=2
  wires:
  Saturation Dynamic/1 -> Goto3/1, Scope2/1
  Sqrt/1 -> Gain1/1, Saturation Dynamic/1  "Iq_ref_nom"
  Iq_ref_nom/1 -> Iq_ref/1
  Square4/1 -> Saturation4/1
  Square3/1 -> Saturation5/1
  Constant1/1 -> Square3/1
  we/1 -> fw gain calculator/1(we)
  Square2/1 -> Sum1/2
  Sum/1 -> Sum1/1  "Vs"
  Constant2/1 -> Square2/1
  Sum3/1 -> Sqrt/1
  Imin/1 -> Saturation Dynamic1/3
  Gain1/1 -> Saturation Dynamic/3
  I_nom/1 -> Product1/1
  Demux/2 -> Square5/1
  Demux/1 -> Square1/1
  Vdq_nonsat/1 -> Demux/1
  Square1/1 -> Sum/1
  Square5/1 -> Sum/2
  From1/1 -> Square4/1
  [Iqref] -> Product1/2
  fw gain calculator/1(Kfw) -> Saturation2/1
  Saturation Dynamic1/1 -> Scope5/1, Id_ref/1, Scope/1, [Idref], Scope1/1
  Sum1/1 -> Product2/2
  Saturation2/1 -> Scope6/1, Product2/1
  Saturation4/1 -> Sum3/2
  Saturation5/1 -> Sum3/1
  Saturation1/1 -> Saturation Dynamic1/2
  Product2/1 -> Gain/1
  Gain/1 -> Saturation1/1
  Imin1/1 -> Saturation Dynamic1/1

== system PMSM_realmodel/phase sync ==
  phi_in : Inport
  wm : Inport  Port=2
  Gain : Gain  Gain=1.5*np/(2*fsw)
  Sum : Sum  Inputs=|++
  phi_out : Outport
  wires:
  wm/1 -> Gain/1
  phi_in/1 -> Sum/1
  Sum/1 -> phi_out/1
  Gain/1 -> Sum/2

== system PMSM_realmodel/w_m -> phi ==
  w_m : Inport
  Constant3 : Constant  Value=2*pi
  Gain1 : Gain  Gain=np
  Integrator2 : Integrator
  Mod : Math  Operator=mod  SignedPower=on
  phi : Outport  VectorParamsAs1DForOutWhenUnconnected=off
  wires:
  Constant3/1 -> Mod/2
  Gain1/1 -> Integrator2/1
  Integrator2/1 -> Mod/1
  Mod/1 -> phi/1  "theta rotor"
  w_m/1 -> Gain1/1

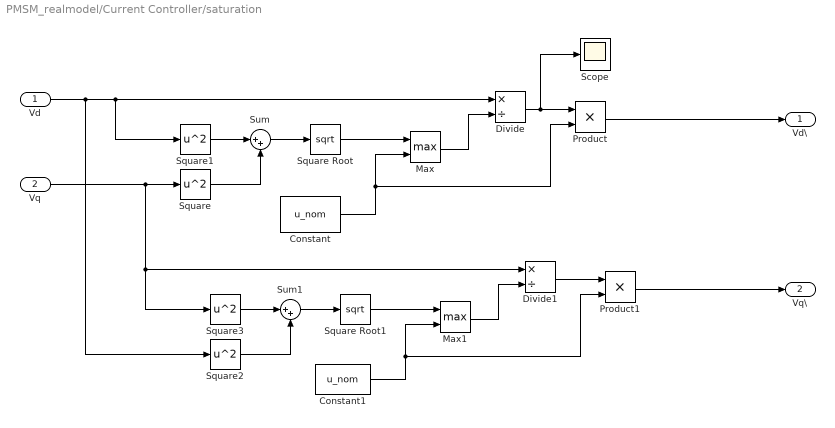
== system PMSM_realmodel/Current Controller/saturation ==
  Vd : Inport
  Vq : Inport  Port=2
  Constant : Constant  Value=u_nom
  Constant1 : Constant  Value=u_nom
  Divide : Product  Inputs=*/
  Divide1 : Product  Inputs=*/
  Max : MinMax  Function=max  Inputs=2
  Max1 : MinMax  Function=max  Inputs=2
  Product : Product
  Product1 : Product
  Scope : Scope
  Square{,1..3} (4 alike) : Math  Operator=square
  Square Root : Sqrt
  Square Root1 : Sqrt
  Sum : Sum  Inputs=|++
  Sum1 : Sum  Inputs=|++
  Vd\ : Outport
  Vq\ : Outport  Port=2
  wires:
  Square1/1 -> Sum/1
  Square/1 -> Sum/2
  Sum/1 -> Square Root/1
  Square Root/1 -> Max/1
  Constant/1 -> Product/2, Max/2
  Max/1 -> Divide/2
  Divide/1 -> Scope/1, Product/1
  Product/1 -> Vd\/1
  Square3/1 -> Sum1/1
  Constant1/1 -> Product1/2, Max1/2
  Square2/1 -> Sum1/2
  Divide1/1 -> Product1/1
  Vd/1 -> Square2/1, Divide/1, Square1/1
  Vq/1 -> Divide1/1, Square3/1, Square/1
  Square Root1/1 -> Max1/1
  Max1/1 -> Divide1/2
  Sum1/1 -> Square Root1/1
  Product1/1 -> Vq\/1

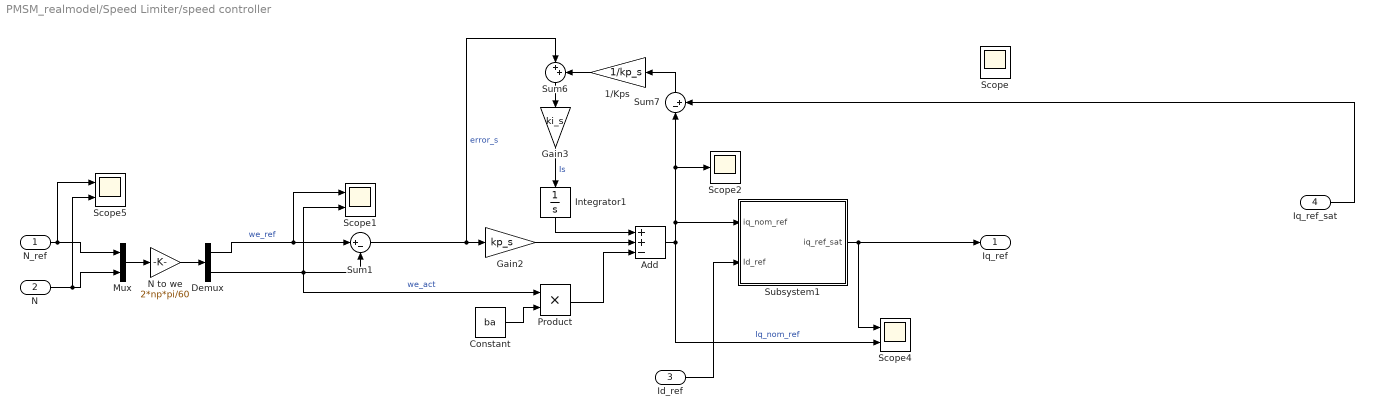
== system PMSM_realmodel/Speed Limiter/speed controller ==
  N_ref : Inport
  N : Inport  Port=2
  Id_ref : Inport  Port=3
  Iq_ref_sat : Inport  Port=4
  1/Kps : Gain  Gain=1/kp_s
  Add : Sum  Inputs=++-
  Constant : Constant  Value=ba
  Demux : Demux  Outputs=2
  Gain2 : Gain  Gain=kp_s
  Gain3 : Gain  Gain=ki_s
  Integrator1 : Integrator
  Mux : Mux  Inputs=2
  N to we : Gain  Gain=2*np*pi/60
  Product : Product
  Scope : Scope
  Scope1 : Scope  NumInputPorts=2
  Scope2 : Scope
  Scope4 : Scope  NumInputPorts=2
  Scope5 : Scope  NumInputPorts=2
  Subsystem1 : Subsystem
  Sum1 : Sum  Inputs=|+-
  Sum6 : Sum  Inputs=|++
  Sum7 : Sum  Inputs=|-+
  Iq_ref : Outport
  wires:
  Sum7/1 -> 1/Kps/1
  Add/1 -> Scope2/1, Sum7/1, Subsystem1/1(iq_nom_ref), Scope4/2  "Iq_nom_ref"
  Gain2/1 -> Add/2
  1/Kps/1 -> Sum6/2
  Sum1/1 -> Gain2/1, Sum6/1  "error_s"
  N_ref/1 -> Scope5/1, Mux/1
  N/1 -> Scope5/2, Mux/2
  Constant/1 -> Product/2
  Gain3/1 -> Integrator1/1  "Is"
  Product/1 -> Add/3
  Demux/1 -> Scope1/1, Sum1/1  "we_ref"
  Demux/2 -> Product/1, Sum1/2, Scope1/2  "we_act"
  Sum6/1 -> Gain3/1
  Subsystem1/1(iq_ref_sat) -> Scope4/1, Iq_ref/1
  Mux/1 -> N to we/1
  N to we/1 -> Demux/1
  Integrator1/1 -> Add/1
  Id_ref/1 -> Subsystem1/2(Id_ref)
  Iq_ref_sat/1 -> Sum7/2

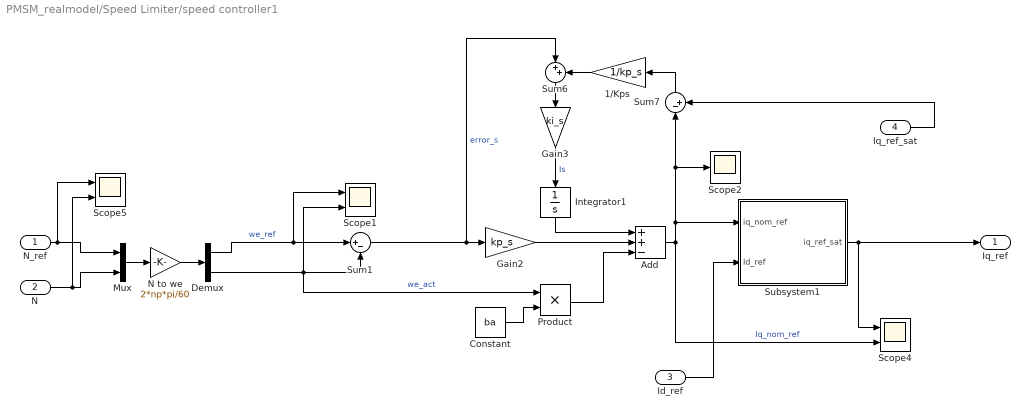
== system PMSM_realmodel/Speed Limiter/speed controller1 ==
  N_ref : Inport
  N : Inport  Port=2
  Id_ref : Inport  Port=3
  Iq_ref_sat : Inport  Port=4
  1/Kps : Gain  Gain=1/kp_s
  Add : Sum  Inputs=++-
  Constant : Constant  Value=ba
  Demux : Demux  Outputs=2
  Gain2 : Gain  Gain=kp_s
  Gain3 : Gain  Gain=ki_s
  Integrator1 : Integrator
  Mux : Mux  Inputs=2
  N to we : Gain  Gain=2*np*pi/60
  Product : Product
  Scope1 : Scope  NumInputPorts=2
  Scope2 : Scope
  Scope4 : Scope  NumInputPorts=2
  Scope5 : Scope  NumInputPorts=2
  Subsystem1 : Subsystem
  Sum1 : Sum  Inputs=|+-
  Sum6 : Sum  Inputs=|++
  Sum7 : Sum  Inputs=|-+
  Iq_ref : Outport
  wires:
  Id_ref/1 -> Subsystem1/2(Id_ref)
  Integrator1/1 -> Add/1
  N to we/1 -> Demux/1
  Mux/1 -> N to we/1
  Subsystem1/1(iq_ref_sat) -> Iq_ref/1, Scope4/1
  Sum6/1 -> Gain3/1
  Demux/2 -> Scope1/2, Sum1/2, Product/1  "we_act"
  Demux/1 -> Sum1/1, Scope1/1  "we_ref"
  Product/1 -> Add/3
  Gain3/1 -> Integrator1/1  "Is"
  Constant/1 -> Product/2
  N/1 -> Mux/2, Scope5/2
  N_ref/1 -> Mux/1, Scope5/1
  Sum1/1 -> Sum6/1, Gain2/1  "error_s"
  1/Kps/1 -> Sum6/2
  Gain2/1 -> Add/2
  Add/1 -> Scope4/2, Subsystem1/1(iq_nom_ref), Sum7/1, Scope2/1  "Iq_nom_ref"
  Sum7/1 -> 1/Kps/1
  Iq_ref_sat/1 -> Sum7/2

== system PMSM_realmodel/fw controller/fw gain calculator ==
  we : Inport
  Abs : Abs  SaturateOnIntegerOverflow=off
  Constant : Constant  Value=a_fw
  Constant1 : Constant  Value=2*Ld
  Constant2 : Constant  Value=u_nom
  Constant3 : Constant  Value=rpm_nom
  Divide : Product  Inputs=*/
  Max : MinMax  Function=max  Inputs=2
  N to we : Gain  Gain=2*np*pi/60
  Product : Product  Inputs=3
  Scope1 : Scope  NumInputPorts=2
  Scope2 : Scope
  Kfw : Outport
  wires:
  N to we/1 -> Max/1, Scope1/1  "we_max"
  Divide/1 -> Kfw/1, Scope2/1
  Product/1 -> Divide/2
  Constant2/1 -> Product/2
  Max/1 -> Product/3
  Constant/1 -> Divide/1
  Constant1/1 -> Product/1
  Abs/1 -> Scope1/2, Max/2  "we"
  we/1 -> Abs/1
  Constant3/1 -> N to we/1

== system PMSM_realmodel/Speed Limiter/speed controller/Subsystem1 ==
  iq_nom_ref : Inport
  Id_ref : Inport  Port=2
  Add : Sum  Inputs=+-
  Constant : Constant  Value=I_max
  Gain : Gain  Gain=-1
  Saturation Dynamic : simulink/Discontinuities/Saturation Dynamic  OutMin=[]  OutMax=[]  OutDataTypeStr=Inherit: Same as second input  OutDataType=fixdt(1, 16)  OutScaling=2^-10  DoSatur=off
  Scope : Scope
  Square Root : Sqrt
  Square1 : Math  Operator=square
  Square2 : Math  Operator=square
  iq_ref_sat : Outport
  wires:
  Square2/1 -> Add/1
  iq_nom_ref/1 -> Saturation Dynamic/2
  Constant/1 -> Square2/1
  Square1/1 -> Add/2
  Square Root/1 -> Gain/1, Saturation Dynamic/1, Scope/1
  Add/1 -> Square Root/1
  Saturation Dynamic/1 -> iq_ref_sat/1
  Id_ref/1 -> Square1/1
  Gain/1 -> Saturation Dynamic/3

== system PMSM_realmodel/Speed Limiter/speed controller1/Subsystem1 ==
  iq_nom_ref : Inport
  Id_ref : Inport  Port=2
  Add : Sum  Inputs=+-
  Constant : Constant  Value=I_max
  Gain : Gain  Gain=-1
  Saturation Dynamic : simulink/Discontinuities/Saturation Dynamic  OutMin=[]  OutMax=[]  OutDataTypeStr=Inherit: Same as second input  OutDataType=fixdt(1, 16)  OutScaling=2^-10  DoSatur=off
  Scope : Scope
  Square Root : Sqrt
  Square1 : Math  Operator=square
  Square2 : Math  Operator=square
  iq_ref_sat : Outport
  wires:
  Id_ref/1 -> Square1/1
  Saturation Dynamic/1 -> iq_ref_sat/1
  Add/1 -> Square Root/1
  Square Root/1 -> Saturation Dynamic/1, Gain/1, Scope/1
  Square1/1 -> Add/2
  Constant/1 -> Square2/1
  iq_nom_ref/1 -> Saturation Dynamic/2
  Square2/1 -> Add/1
  Gain/1 -> Saturation Dynamic/3
